simulink model "Copy_of_test_PassVeh_acc"  (R2018b)
settings: configuration reference "Physics" (kept outside this file)
model workspace (MAT data in the model file):
  m = 1000
libraries: simulink x1
settings Model: DataDictionary=test_PassengerVehicle.sldd  PauseTimes=9.280  Creator=wischnewski  LastModifiedBy=Michael

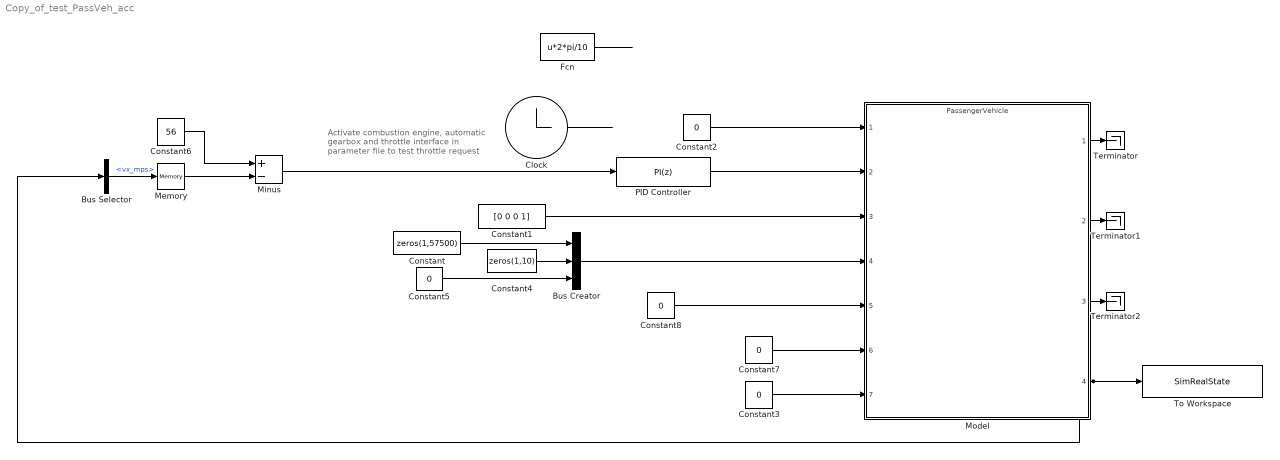
== system Copy_of_test_PassVeh_acc ==
  note: Activate combustion engine, automatic gearbox and throttle interface in parameter file to test throttle request
  Bus Creator : BusCreator  Inputs=3  OutDataTypeStr=Bus: tpamapReference
  Bus Selector : BusSelector  OutputSignals=vx_mps
  Clock : Clock
  Constant : Constant  Value=zeros(1,57500)
  Constant1 : Constant  Value=[0 0 0 1]
  Constant{2..3,5,7..8} (5 alike) : Constant  Value=0
  Constant4 : Constant  Value=zeros(1,10)
  Constant6 : Constant  Value=56
  Fcn : Fcn  Expr=u*2*pi/10
  Memory : Memory
  Minus : Sum  Inputs=+-
  Model : ModelReference  ModelNameDialog=PassengerVehicle.slx  SimulationMode=Normal  ModelReferenceVersion=1.936
  PID Controller : simulink/Continuous/PID Controller  Controller=PI  Form=Parallel  TimeDomain=Discrete-time  SampleTime=-1  IntegratorMethod=Forward Euler  FilterMethod=Forward Euler  ControllerParametersSource=internal  P=1000  I=10  D=0  UseFilter=on  N=100  TunerSelectOption=Transfer Function Based (PID Tuner App)  InitialConditionSource=internal  InitialConditionForIntegrator=0  InitialConditionForFilter=0  DifferentiatorICPrevScaledInput=0  ExternalReset=none  TrackingMode=off  Kt=1  LimitOutput=on  UpperSaturationLimit=4000  LowerSaturationLimit=0  LinearizeAsGain=on  AntiWindupMode=none  Kb=1  POutMin=[]  POutMax=[]  IOutMin=[]  IOutMax=[]  DOutMin=[]  DOutMax=[]  NOutMin=[]  NOutMax=[]  SumOutMin=[]  SumOutMax=[]  SaturationOutMin=[]  SaturationOutMax=[]  PParamMin=[]  PParamMax=[]  IParamMin=[]  IParamMax=[]  DParamMin=[]  DParamMax=[]  NParamMin=[]  NParamMax=[]  KbParamMin=[]  KbParamMax=[]  KtParamMin=[]  KtParamMax=[]  KbOutMin=[]  KbOutMax=[]  KtOutMin=[]  KtOutMax=[]  IntegratorOutMin=[]  IntegratorOutMax=[]  FilterOutMin=[]  FilterOutMax=[]  SumI1OutMin=[]  SumI1OutMax=[]  SumI2OutMin=[]  SumI2OutMax=[]  SumI3OutMin=[]  SumI3OutMax=[]  SumI4OutMin=[]  SumI4OutMax=[]  SumDOutMin=[]  SumDOutMax=[]  DifferentiatorOutMin=[]  DifferentiatorOutMax=[]  FilterDiffOutCoefMin=[]  FilterDiffOutCoefMax=[]  ReciprocalOutMin=[]  ReciprocalOutMax=[]  SumDenOutMin=[]  SumDenOutMax=[]  SumNumOutMin=[]  SumNumOutMax=[]  DivideOutMin=[]  DivideOutMax=[]  IntegratorContinuousStateAttributes=''  IntegratorStateMustResolveToSignalObject=off  IntegratorRTWStateStorageClass=Auto  FilterContinuousStateAttributes=''  FilterStateMustResolveToSignalObject=off  FilterRTWStateStorageClass=Auto  ParallelPVariant=InternalParameters  IdealPVariant=Disabled  IVariant=InternalParameters  DVariant=Disabled  IntegratorVariant=Discrete  SatVariant=Enabled  AWVariant=Passthrough  PCopyVariant=Disabled  TRVariant=Disabled  FdbkBlocksVariant=Forward  IdealPFdbkVariant=Disabled  SatFdbkVariant=Disabled  DerivativeFilterVariant=Disabled  NVariant=Disabled  NCopyVariant=Disabled_SignalSpec  FilterICVariant=Disabled  IntegratorICVariant=InternalICs  ExternalResetVariant=Disabled  TRSumVariant=Passthrough  SumFdbkVariant=Disabled  SumVariant=Sum_PI
  Terminator : Terminator
  Terminator1 : Terminator
  Terminator2 : Terminator
  To Workspace : ToWorkspace  VariableName=SimRealState  SaveFormat=Timeseries  SampleTime=-1
  wires:
  Bus Creator/1 -> Model/4
  Constant1/1 -> Model/3
  Fcn/1 -> ?
  Model/1 -> Terminator/1
  Model/3 -> Terminator2/1
  Model/2 -> Terminator1/1
  PID Controller/1 -> Model/2
  Constant/1 -> Bus Creator/1
  Constant4/1 -> Bus Creator/2
  Constant5/1 -> Bus Creator/3
  Model/4 -> To Workspace/1, Bus Selector/1
  Bus Selector/1 -> Memory/1  "<vx_mps>"
  Constant6/1 -> Minus/1
  Memory/1 -> Minus/2
  Minus/1 -> PID Controller/1
  Constant7/1 -> Model/6
  Constant3/1 -> Model/7
  Constant8/1 -> Model/5
  Clock/1 -> ?
  Constant2/1 -> Model/1
